simulink model "Traction_invertor"  (R2024b)
settings: Solver=VariableStepAuto  StartTime=0.0  StopTime=1  RelTol=1e-3
libraries: spsMosfetLib x6, spsVoltageMeasurementLib x6, spsCurrentMeasurementLib x3, spsSeriesRLCBranchLib x3, spsDCVoltageSourceLib x1, simulink x1, sps_lib x1
settings Model: Creator=Jayde  LastModifiedBy=Jayde

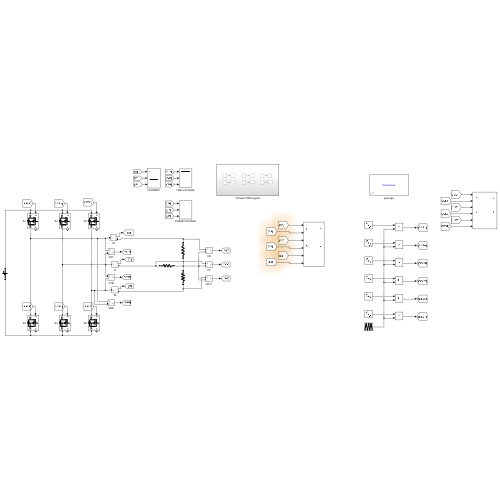
[thumbnail: Simulink's stored preview of the top-level diagram]
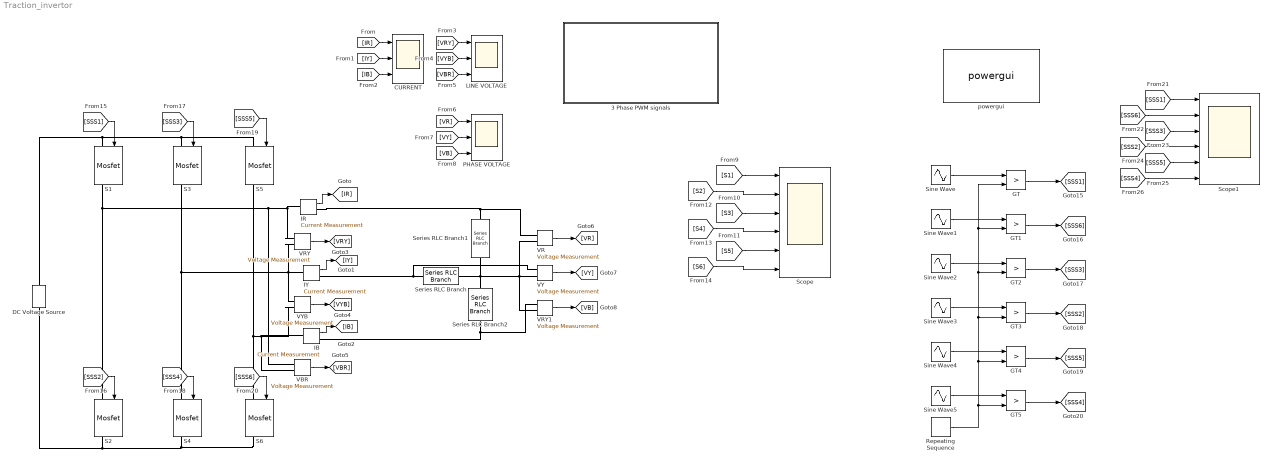
== system Traction_invertor ==
  3 Phase PWM signals : Subsystem
  CURRENT : Scope  NumInputPorts=3
  DC Voltage Source : spsDCVoltageSourceLib/DC Voltage Source  Amplitude=100  Measurements=None
  GT{,1..5} (6 alike) : RelationalOperator  Operator=>  OutDataTypeStr=boolean  RndMeth=Simplest  InputSameDT=off
  IB : spsCurrentMeasurementLib/Current Measurement  PhasorSimulation=off  OutputType=Complex  PSBequivalent=0
  IR : spsCurrentMeasurementLib/Current Measurement  PhasorSimulation=off  OutputType=Complex  PSBequivalent=0
  IY : spsCurrentMeasurementLib/Current Measurement  PhasorSimulation=off  OutputType=Complex  PSBequivalent=0
  LINE VOLTAGE : Scope  NumInputPorts=3
  PHASE VOLTAGE : Scope  NumInputPorts=3
  Repeating Sequence : simulink/Sources/Repeating Sequence  rep_seq_t=[0 0.02/40 0.02/20]  rep_seq_y=[0 2 0]
  S{1..6} (6 alike) : spsMosfetLib/Mosfet  Ron=0.1  Lon=0  Rd=0.01  Vfd=0  IC=0  Rs=1e5  Cs=inf  Measurements=on
  Scope : Scope  NumInputPorts=6
  Scope1 : Scope  NumInputPorts=6
  Series RLC Branch : spsSeriesRLCBranchLib/Series RLC Branch  LConnTagsString=__new0  RConnTagsString=__new0  BranchType=R  Resistance=1  Inductance=1e-3  SetiL0=off  InitialCurrent=0  Capacitance=1e-6  Setx0=off  InitialVoltage=0  Measurements=None
  Series RLC Branch1 : spsSeriesRLCBranchLib/Series RLC Branch  LConnTagsString=__new0  RConnTagsString=__new0  BranchType=R  Resistance=1  Inductance=1e-3  SetiL0=off  InitialCurrent=0  Capacitance=1e-6  Setx0=off  InitialVoltage=0  Measurements=None
  Series RLC Branch2 : spsSeriesRLCBranchLib/Series RLC Branch  LConnTagsString=__new0  RConnTagsString=__new0  BranchType=R  Resistance=1  Inductance=1e-3  SetiL0=off  InitialCurrent=0  Capacitance=1e-6  Setx0=off  InitialVoltage=0  Measurements=None
  Sine Wave : Sin  Frequency=2*pi*50  SampleTime=0
  Sine Wave1 : Sin  Frequency=2*pi*50  Phase=60*(pi/180)  SampleTime=0
  Sine Wave2 : Sin  Frequency=2*pi*50  Phase=120*(pi/360)  SampleTime=0
  Sine Wave3 : Sin  Frequency=2*pi*50  Phase=180*(pi/360)  SampleTime=0
  Sine Wave4 : Sin  Frequency=2*pi*50  Phase=240*(pi/360)  SampleTime=0
  Sine Wave5 : Sin  Frequency=2*pi*50  Phase=300*(pi/360)  SampleTime=0
  VBR : spsVoltageMeasurementLib/Voltage Measurement  PhasorSimulation=off  OutputType=Complex  PSBequivalent=0
  VR : spsVoltageMeasurementLib/Voltage Measurement  PhasorSimulation=off  OutputType=Complex  PSBequivalent=0
  VRY : spsVoltageMeasurementLib/Voltage Measurement  PhasorSimulation=off  OutputType=Complex  PSBequivalent=0
  VRY1 : spsVoltageMeasurementLib/Voltage Measurement  PhasorSimulation=off  OutputType=Complex  PSBequivalent=0
  VY : spsVoltageMeasurementLib/Voltage Measurement  PhasorSimulation=off  OutputType=Complex  PSBequivalent=0
  VYB : spsVoltageMeasurementLib/Voltage Measurement  PhasorSimulation=off  OutputType=Complex  PSBequivalent=0
  powergui : sps_lib/powergui  Priority=1  SimulationMode=Continuous  SampleTime=50e-6  frequency=60  Iterations=50  frequencyindice=0  Pbase=100e6  ErrMax=1e-4  UnitsV=kV  UnitsW=MW  buscounter=0  FunctionMessages=off  echomessages=off  EnableUseOfTLC=off  CurrentSourceSwitches=off  DisableSnubberDevices=off  DisableRonSwitches=off  DisableVfSwitches=off  DisplayEquations=off  AutomaticDiscreteSolvers=off  SolverType=Tustin/Backward Euler (TBE)  Interpol=off  ExternalGateDelay=off  methode=off  Ts=100  x0status=blocks  SPID=on  SwTol=0  HookPort=off  NonlinearTolerance=1e-4  nMaxIteration=100  ContinueOnMaxIteration=off  RestoreLinks=warning  ResistiveCurrentMeasurement=off  Frange=[0:2:500]  Ylog=off  Xlog=on  ShowGrid=off  save=off  variable=ZData  structure=0  ZoomFFT=off  StartTime=0.0  cycles=1  DisplayStyle=1  fundamental=60  FreqAxis=off  MaxFrequency=1000  frequencyindicesteady=1  RmsSteady=1  display=off
  wires:
  IR/1 -> [IR]
  IY/1 -> [IY]
  IB/1 -> [IB]
  VRY/1 -> [VRY]
  VYB/1 -> [VYB]
  VBR/1 -> [VBR]
  VR/1 -> [VR]
  VY/1 -> [VY]
  VRY1/1 -> [VB]
  [IR] -> CURRENT/1
  [IY] -> CURRENT/2
  [IB] -> CURRENT/3
  [VBR] -> LINE VOLTAGE/3
  [VYB] -> LINE VOLTAGE/2
  [VRY] -> LINE VOLTAGE/1
  [VB] -> PHASE VOLTAGE/3
  [VY] -> PHASE VOLTAGE/2
  [VR] -> PHASE VOLTAGE/1
  [S1] -> Scope/1
  [S3] -> Scope/3
  [S5] -> Scope/5
  [S2] -> Scope/2
  [S4] -> Scope/4
  [S6] -> Scope/6
  [SSS1] -> S1/1
  [SSS2] -> S2/1
  [SSS3] -> S3/1
  [SSS4] -> S4/1
  [SSS5] -> S5/1
  [SSS6] -> S6/1
  Sine Wave/1 -> GT/1
  GT/1 -> [SSS1]
  Sine Wave1/1 -> GT1/1
  GT1/1 -> [SSS6]
  Sine Wave2/1 -> GT2/1
  GT2/1 -> [SSS3]
  Sine Wave3/1 -> GT3/1
  GT3/1 -> [SSS2]
  Sine Wave4/1 -> GT4/1
  GT4/1 -> [SSS5]
  Sine Wave5/1 -> GT5/1
  GT5/1 -> [SSS4]
  [SSS1] -> Scope1/1
  [SSS6] -> Scope1/2
  [SSS3] -> Scope1/3
  [SSS2] -> Scope1/4
  [SSS5] -> Scope1/5
  [SSS4] -> Scope1/6
  Repeating Sequence/1 -> GT5/2, GT3/2, GT2/2, GT1/2, GT/2, GT4/2
  connections:
  S1/RConn1 -- S2/LConn1 -- VBR/LConn1 -- VRY/LConn1 -- IR/LConn1
  S4/LConn1 -- S3/RConn1 -- IY/LConn1 -- VRY/LConn2 -- VYB/LConn1
  S5/RConn1 -- VYB/LConn2 -- IB/LConn1 -- VBR/LConn2 -- S6/LConn1
  S3/LConn1 -- S5/LConn1 -- DC Voltage Source/RConn1 -- S1/LConn1
  S2/RConn1 -- S6/RConn1 -- S4/RConn1 -- DC Voltage Source/LConn1
  IR/RConn1 -- VR/LConn1 -- Series RLC Branch1/LConn1
  IB/RConn1 -- VRY1/LConn1 -- Series RLC Branch2/RConn1
  Series RLC Branch/LConn1 -- VY/LConn1 -- IY/RConn1
  Series RLC Branch/RConn1 -- VY/LConn2 -- VRY1/LConn2 -- VR/LConn2 -- Series RLC Branch1/RConn1 -- Series RLC Branch2/LConn1

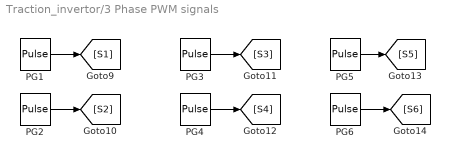
== system Traction_invertor/3 Phase PWM signals ==
  PG1 : DiscretePulseGenerator  PulseType=Time based  Period=0.02  PulseWidth=50
  PG2 : DiscretePulseGenerator  PulseType=Time based  Period=0.02  PulseWidth=50  PhaseDelay=180*0.02/360
  PG3 : DiscretePulseGenerator  PulseType=Time based  Period=0.02  PulseWidth=50  PhaseDelay=120*0.02/360
  PG4 : DiscretePulseGenerator  PulseType=Time based  Period=0.02  PulseWidth=50  PhaseDelay=300*0.02/360
  PG5 : DiscretePulseGenerator  PulseType=Time based  Period=0.02  PulseWidth=50  PhaseDelay=240*0.02/360
  PG6 : DiscretePulseGenerator  PulseType=Time based  Period=0.02  PulseWidth=50  PhaseDelay=60*0.02/360
  wires:
  PG3/1 -> [S3]
  PG4/1 -> [S4]
  PG2/1 -> [S2]
  PG1/1 -> [S1]
  PG6/1 -> [S6]
  PG5/1 -> [S5]
